simulink model "DCMotorModel"  (Simulink 7.8)
settings: Solver=ode23  StartTime=0.0  StopTime=3.0  RelTol=1e-3
settings Model: Creator=maen  LastModifiedBy=evgenov
settings DebuggingCC: FcnCallInpInsideContextMsg=Use local settings

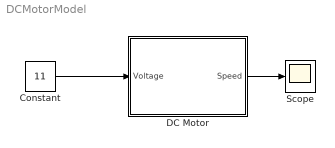
== system DCMotorModel ==
  Constant : Constant  Value=11
  DC Motor : Subsystem
  Scope : Scope
      settings: YMin=1.5  YMax=5.25  SampleInput=on
  wires:
  Constant/1 -> DC Motor/1(Voltage)
  DC Motor/1(" Speed") -> Scope/1

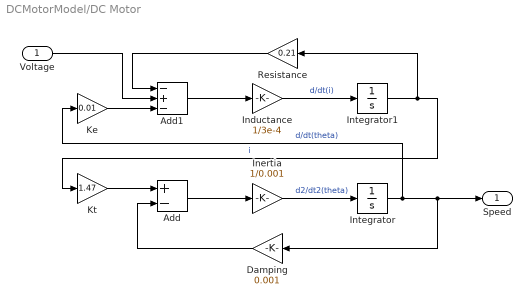
== system DCMotorModel/DC Motor ==
  Voltage : Inport
  Add : Sum  Inputs=+-
  Add1 : Sum  Inputs=-+-
  Damping : Gain  Gain=0.001
  Inductance : Gain  Gain=1/3e-4
  Inertia : Gain  Gain=1/0.001
  Integrator : Integrator
  Integrator1 : Integrator
  Ke : Gain  Gain=0.01
  Kt : Gain  Gain=1.47
  Resistance : Gain  Gain=0.21
  " Speed" : Outport
  wires:
  Integrator1/1 -> Kt/1, Resistance/1  "i"
  Inductance/1 -> Integrator1/1  "d/dt(i)"
  Inertia/1 -> Integrator/1  "d2/dt2(theta)"
  Integrator/1 -> Ke/1, Damping/1, " Speed"/1  "d/dt(theta)"
  Add1/1 -> Inductance/1
  Add/1 -> Inertia/1
  Damping/1 -> Add/2
  Kt/1 -> Add/1
  Resistance/1 -> Add1/1
  Ke/1 -> Add1/3
  Voltage/1 -> Add1/2
